simulink model "SingleLeg_R2013a"  (R2013a)
settings: Solver=FixedStepDiscrete  StartTime=0.0  StopTime=inf  FixedStep=0.001  RelTol=1e-3
libraries: xpcethercatlib x30, dspswit3 x1
settings Model: BufferReuse=off  Creator=bgbuss  LastModifiedBy=bgbuss
settings OptimizationCC: BlockReduction=off  OptimizeBlockIOStorage=off  BufferReuse=off  ExpressionFolding=off  LocalBlockOutputs=off
settings DebuggingCC: UnderspecifiedInitializationDetection=Simplified
settings HardwareCC: ProdIntDivRoundTo=Zero  ProdEndianess=LittleEndian  ProdHWDeviceType=Generic->32-bit x86 compatible
settings RTWCC: SystemTargetFile=xpctarget.tlc  TemplateMakefile=xpc_default_tmf  Description=xPC Target  ProcessScript=xpctarget_make_rtw_hook  RTWCompilerOptimization=On
settings CodeAppCC: MATLABSourceComments=on
settings xpcTargetCC: TargetFcnLib=ansi_tfl_table_tmw.mat  CodeReplacementLibrary=XPC_BLAS  ParMdlRefBuildCompliant=on  ConcurrentExecutionCompliant=on  CombineSignalStateStructs=off  MATLABClassNameForMDSCustomization=xpcAperiodicCustomization  GRTInterface=on  GenerateAllocFcn=off  RL32LogBufSizeModifier=100000000  xPCTaskExecutionProfile=off  xPCRL32EventNumber=5000  xPCisModelTimeout=off  xPCModelTimeoutSecs=20  xPCLoadParamSetFile=off  xPCConcurrentTasks=off  xPCEnableSFAnimation=off

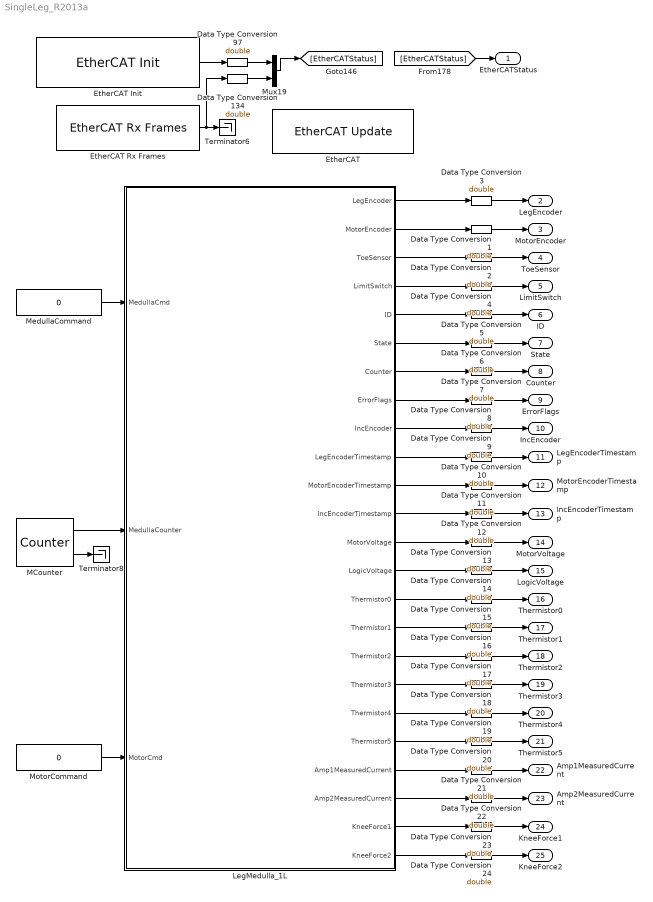
== system SingleLeg_R2013a ==
  Data Type Conversion{1..24,97,134} (26 alike) : DataTypeConversion  OutDataTypeStr=double
  EtherCAT : xpcethercatlib/EtherCAT Update   Priority=4  device_id=0  task_id_list=[1]  task_rates=[1]  task_priorities=[1500]
  "EtherCAT Init " : xpcethercatlib/EtherCAT Init   Priority=0  config_file='SingleLeg-eni.xml'  device_id=0  pci_bus=10  pci_slot=0  enaDC=on  errRptLevel=0  sample_time=-1
  EtherCAT Rx Frames : xpcethercatlib/EtherCAT Rx Frames   Priority=1  device_id=0  sample_time=0
  LegMedulla_1L : Subsystem
  MCounter : dspswit3/Counter  Direction=Up  CountEvent=Free running  CounterSize=User defined  MaxCount=65535  InitialCount=0  Output=Count and Hit  HitValue=32  ResetInput=off  SamplesPerFrame=1  Ts=.001  CntDtype=double  HitDtype=Logical
  MedullaCommand : Constant  Value=0
  MotorCommand : Constant  Value=0
  Mux19 : Mux  Inputs=2
  Terminator6 : Terminator
  Terminator8 : Terminator
  EtherCATStatus : Outport
  LegEncoder : Outport  Port=2
  MotorEncoder : Outport  Port=3
  ToeSensor : Outport  Port=4
  LimitSwitch : Outport  Port=5
  ID : Outport  Port=6
  State : Outport  Port=7
  Counter : Outport  Port=8
  ErrorFlags : Outport  Port=9
  IncEncoder : Outport  Port=10
  LegEncoderTimestamp : Outport  Port=11
  MotorEncoderTimestamp : Outport  Port=12
  IncEncoderTimestamp : Outport  Port=13
  MotorVoltage : Outport  Port=14
  LogicVoltage : Outport  Port=15
  Thermistor0 : Outport  Port=16
  Thermistor1 : Outport  Port=17
  Thermistor2 : Outport  Port=18
  Thermistor3 : Outport  Port=19
  Thermistor4 : Outport  Port=20
  Thermistor5 : Outport  Port=21
  Amp1MeasuredCurrent : Outport  Port=22
  Amp2MeasuredCurrent : Outport  Port=23
  KneeForce1 : Outport  Port=24
  KneeForce2 : Outport  Port=25
  wires:
  Data Type Conversion3/1 -> LegEncoder/1
  [EtherCATStatus] -> EtherCATStatus/1
  Mux19/1 -> [EtherCATStatus]
  "EtherCAT Init "/1 -> Data Type Conversion97/1
  LegMedulla_1L/2(MotorEncoder) -> Data Type Conversion1/1
  LegMedulla_1L/3(ToeSensor) -> Data Type Conversion2/1
  LegMedulla_1L/4(LimitSwitch) -> Data Type Conversion4/1
  LegMedulla_1L/5(ID) -> Data Type Conversion5/1
  LegMedulla_1L/6(State) -> Data Type Conversion6/1
  LegMedulla_1L/7(Counter) -> Data Type Conversion7/1
  LegMedulla_1L/8(ErrorFlags) -> Data Type Conversion8/1
  LegMedulla_1L/9(IncEncoder) -> Data Type Conversion9/1
  LegMedulla_1L/10(LegEncoderTimestamp) -> Data Type Conversion10/1
  LegMedulla_1L/11(MotorEncoderTimestamp) -> Data Type Conversion11/1
  LegMedulla_1L/12(IncEncoderTimestamp) -> Data Type Conversion12/1
  LegMedulla_1L/13(MotorVoltage) -> Data Type Conversion13/1
  LegMedulla_1L/14(LogicVoltage) -> Data Type Conversion14/1
  LegMedulla_1L/15(Thermistor0) -> Data Type Conversion15/1
  LegMedulla_1L/16(Thermistor1) -> Data Type Conversion16/1
  LegMedulla_1L/17(Thermistor2) -> Data Type Conversion17/1
  LegMedulla_1L/18(Thermistor3) -> Data Type Conversion18/1
  LegMedulla_1L/19(Thermistor4) -> Data Type Conversion19/1
  LegMedulla_1L/20(Thermistor5) -> Data Type Conversion20/1
  LegMedulla_1L/21(Amp1MeasuredCurrent) -> Data Type Conversion21/1
  LegMedulla_1L/22(Amp2MeasuredCurrent) -> Data Type Conversion22/1
  LegMedulla_1L/23(KneeForce1) -> Data Type Conversion23/1
  LegMedulla_1L/24(KneeForce2) -> Data Type Conversion24/1
  EtherCAT Rx Frames/1 -> Data Type Conversion134/1, Terminator6/1
  MCounter/2 -> Terminator8/1
  LegMedulla_1L/1(LegEncoder) -> Data Type Conversion3/1
  Data Type Conversion5/1 -> ID/1
  Data Type Conversion6/1 -> State/1
  Data Type Conversion7/1 -> Counter/1
  Data Type Conversion8/1 -> ErrorFlags/1
  Data Type Conversion9/1 -> IncEncoder/1
  Data Type Conversion10/1 -> LegEncoderTimestamp/1
  Data Type Conversion11/1 -> MotorEncoderTimestamp/1
  Data Type Conversion12/1 -> IncEncoderTimestamp/1
  Data Type Conversion13/1 -> MotorVoltage/1
  Data Type Conversion14/1 -> LogicVoltage/1
  Data Type Conversion15/1 -> Thermistor0/1
  Data Type Conversion16/1 -> Thermistor1/1
  Data Type Conversion17/1 -> Thermistor2/1
  Data Type Conversion18/1 -> Thermistor3/1
  Data Type Conversion19/1 -> Thermistor4/1
  Data Type Conversion20/1 -> Thermistor5/1
  Data Type Conversion21/1 -> Amp1MeasuredCurrent/1
  Data Type Conversion22/1 -> Amp2MeasuredCurrent/1
  Data Type Conversion23/1 -> KneeForce1/1
  Data Type Conversion24/1 -> KneeForce2/1
  MCounter/1 -> LegMedulla_1L/2(MedullaCounter)
  MedullaCommand/1 -> LegMedulla_1L/1(MedullaCmd)
  MotorCommand/1 -> LegMedulla_1L/3(MotorCmd)
  Data Type Conversion2/1 -> ToeSensor/1
  Data Type Conversion4/1 -> LimitSwitch/1
  Data Type Conversion1/1 -> MotorEncoder/1
  Data Type Conversion97/1 -> Mux19/1
  Data Type Conversion134/1 -> Mux19/2

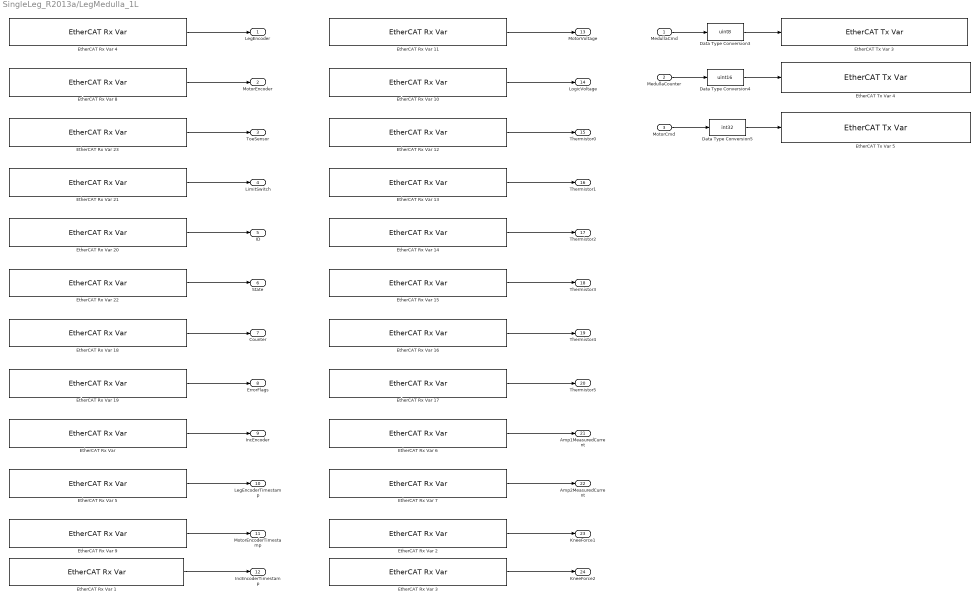
== system SingleLeg_R2013a/LegMedulla_1L ==
  MedullaCmd : Inport
  MedullaCounter : Inport  Port=2
  MotorCmd : Inport  Port=3
  Data Type Conversion3 : DataTypeConversion  OutDataTypeStr=uint8
  Data Type Conversion4 : DataTypeConversion  OutDataTypeStr=uint16
  Data Type Conversion5 : DataTypeConversion  OutDataTypeStr=int32
  "EtherCAT Rx Var " : xpcethercatlib/EtherCAT Rx Var   Priority=2  sig_name=Box 1 (ATRIAS 2.1 Leg (Medulla 1.5)).Incremental Encoder.Incremental Encoder  sig_offset=744  sig_type=uint16  type_size=16  sig_dim=1  device_id=0  sample_time=0.001000
  EtherCAT Rx Var 1 : xpcethercatlib/EtherCAT Rx Var   Priority=2  sig_name=Box 1 (ATRIAS 2.1 Leg (Medulla 1.5)).Incremental Encoder.Incremental Encoder Timestamp  sig_offset=760  sig_type=uint16  type_size=16  sig_dim=1  device_id=0  sample_time=0.001000
  EtherCAT Rx Var 10 : xpcethercatlib/EtherCAT Rx Var   Priority=2  sig_name=Box 1 (ATRIAS 2.1 Leg (Medulla 1.5)).Power.Logic Voltage  sig_offset=792  sig_type=uint16  type_size=16  sig_dim=1  device_id=0  sample_time=0.001000
  EtherCAT Rx Var 11 : xpcethercatlib/EtherCAT Rx Var   Priority=2  sig_name=Box 1 (ATRIAS 2.1 Leg (Medulla 1.5)).Power.Motor Voltage  sig_offset=776  sig_type=uint16  type_size=16  sig_dim=1  device_id=0  sample_time=0.001000
  EtherCAT Rx Var 12 : xpcethercatlib/EtherCAT Rx Var   Priority=2  sig_name=Box 1 (ATRIAS 2.1 Leg (Medulla 1.5)).Thermistors.Thermistor 0  sig_offset=808  sig_type=uint16  type_size=16  sig_dim=1  device_id=0  sample_time=0.001000
  EtherCAT Rx Var 13 : xpcethercatlib/EtherCAT Rx Var   Priority=2  sig_name=Box 1 (ATRIAS 2.1 Leg (Medulla 1.5)).Thermistors.Thermistor 1  sig_offset=824  sig_type=uint16  type_size=16  sig_dim=1  device_id=0  sample_time=0.001000
  EtherCAT Rx Var 14 : xpcethercatlib/EtherCAT Rx Var   Priority=2  sig_name=Box 1 (ATRIAS 2.1 Leg (Medulla 1.5)).Thermistors.Thermistor 2  sig_offset=840  sig_type=uint16  type_size=16  sig_dim=1  device_id=0  sample_time=0.001000
  EtherCAT Rx Var 15 : xpcethercatlib/EtherCAT Rx Var   Priority=2  sig_name=Box 1 (ATRIAS 2.1 Leg (Medulla 1.5)).Thermistors.Thermistor 3  sig_offset=856  sig_type=uint16  type_size=16  sig_dim=1  device_id=0  sample_time=0.001000
  EtherCAT Rx Var 16 : xpcethercatlib/EtherCAT Rx Var   Priority=2  sig_name=Box 1 (ATRIAS 2.1 Leg (Medulla 1.5)).Thermistors.Thermistor 4  sig_offset=872  sig_type=uint16  type_size=16  sig_dim=1  device_id=0  sample_time=0.001000
  EtherCAT Rx Var 17 : xpcethercatlib/EtherCAT Rx Var   Priority=2  sig_name=Box 1 (ATRIAS 2.1 Leg (Medulla 1.5)).Thermistors.Thermistor 5  sig_offset=888  sig_type=uint16  type_size=16  sig_dim=1  device_id=0  sample_time=0.001000
  EtherCAT Rx Var 18 : xpcethercatlib/EtherCAT Rx Var   Priority=2  sig_name=Box 1 (ATRIAS 2.1 Leg (Medulla 1.5)).uController Status.Counter  sig_offset=608  sig_type=uint8  type_size=8  sig_dim=1  device_id=0  sample_time=0.001000
  EtherCAT Rx Var 19 : xpcethercatlib/EtherCAT Rx Var   Priority=2  sig_name=Box 1 (ATRIAS 2.1 Leg (Medulla 1.5)).uController Status.Error Flags  sig_offset=616  sig_type=uint8  type_size=8  sig_dim=1  device_id=0  sample_time=0.001000
  EtherCAT Rx Var 2 : xpcethercatlib/EtherCAT Rx Var   Priority=2  sig_name=Box 1 (ATRIAS 2.1 Leg (Medulla 1.5)).Knee Force.Knee Force 1  sig_offset=936  sig_type=uint16  type_size=16  sig_dim=1  device_id=0  sample_time=0.001000
  EtherCAT Rx Var 20 : xpcethercatlib/EtherCAT Rx Var   Priority=2  sig_name=Box 1 (ATRIAS 2.1 Leg (Medulla 1.5)).uController Status.ID  sig_offset=592  sig_type=uint8  type_size=8  sig_dim=1  device_id=0  sample_time=0.001000
  EtherCAT Rx Var 21 : xpcethercatlib/EtherCAT Rx Var   Priority=2  sig_name=Box 1 (ATRIAS 2.1 Leg (Medulla 1.5)).uController Status.Limit Switch  sig_offset=624  sig_type=uint8  type_size=8  sig_dim=1  device_id=0  sample_time=0.001000
  EtherCAT Rx Var 22 : xpcethercatlib/EtherCAT Rx Var   Priority=2  sig_name=Box 1 (ATRIAS 2.1 Leg (Medulla 1.5)).uController Status.State  sig_offset=600  sig_type=uint8  type_size=8  sig_dim=1  device_id=0  sample_time=0.001000
  EtherCAT Rx Var 23 : xpcethercatlib/EtherCAT Rx Var   Priority=2  sig_name=Box 1 (ATRIAS 2.1 Leg (Medulla 1.5)).uController Status.Toe Sensor  sig_offset=632  sig_type=uint16  type_size=16  sig_dim=1  device_id=0  sample_time=0.001000
  EtherCAT Rx Var 3 : xpcethercatlib/EtherCAT Rx Var   Priority=2  sig_name=Box 1 (ATRIAS 2.1 Leg (Medulla 1.5)).Knee Force.Knee Force 2  sig_offset=952  sig_type=uint16  type_size=16  sig_dim=1  device_id=0  sample_time=0.001000
  EtherCAT Rx Var 4 : xpcethercatlib/EtherCAT Rx Var   Priority=2  sig_name=Box 1 (ATRIAS 2.1 Leg (Medulla 1.5)).Leg Encoder.Leg Encoder  sig_offset=696  sig_type=uint32  type_size=32  sig_dim=1  device_id=0  sample_time=0.001000
  EtherCAT Rx Var 5 : xpcethercatlib/EtherCAT Rx Var   Priority=2  sig_name=Box 1 (ATRIAS 2.1 Leg (Medulla 1.5)).Leg Encoder.Leg Encoder Timestamp  sig_offset=728  sig_type=uint16  type_size=16  sig_dim=1  device_id=0  sample_time=0.001000
  EtherCAT Rx Var 6 : xpcethercatlib/EtherCAT Rx Var   Priority=2  sig_name=Box 1 (ATRIAS 2.1 Leg (Medulla 1.5)).Measured Current.Amp 1 Measured Current  sig_offset=904  sig_type=int16  type_size=16  sig_dim=1  device_id=0  sample_time=0.001000
  EtherCAT Rx Var 7 : xpcethercatlib/EtherCAT Rx Var   Priority=2  sig_name=Box 1 (ATRIAS 2.1 Leg (Medulla 1.5)).Measured Current.Amp 2 Measured Current  sig_offset=920  sig_type=int16  type_size=16  sig_dim=1  device_id=0  sample_time=0.001000
  EtherCAT Rx Var 8 : xpcethercatlib/EtherCAT Rx Var   Priority=2  sig_name=Box 1 (ATRIAS 2.1 Leg (Medulla 1.5)).Motor Encoder.Motor Encoder  sig_offset=648  sig_type=uint32  type_size=32  sig_dim=1  device_id=0  sample_time=0.001000
  EtherCAT Rx Var 9 : xpcethercatlib/EtherCAT Rx Var   Priority=2  sig_name=Box 1 (ATRIAS 2.1 Leg (Medulla 1.5)).Motor Encoder.Motor Encoder Timestamp  sig_offset=680  sig_type=uint16  type_size=16  sig_dim=1  device_id=0  sample_time=0.001000
  EtherCAT Tx Var 3 : xpcethercatlib/EtherCAT Tx Var   Priority=3  sig_name=Box 1 (ATRIAS 2.1 Leg (Medulla 1.5)).uControllerInput.Command  sig_offset=592  sig_type=uint8  type_size=8  sig_dim=1  device_id=0  sample_time=0.001000
  EtherCAT Tx Var 4 : xpcethercatlib/EtherCAT Tx Var   Priority=3  sig_name=Box 1 (ATRIAS 2.1 Leg (Medulla 1.5)).uControllerInput.Counter  sig_offset=600  sig_type=uint16  type_size=16  sig_dim=1  device_id=0  sample_time=0.001000
  EtherCAT Tx Var 5 : xpcethercatlib/EtherCAT Tx Var   Priority=3  sig_name=Box 1 (ATRIAS 2.1 Leg (Medulla 1.5)).uControllerInput.Motor Current  sig_offset=616  sig_type=int32  type_size=32  sig_dim=1  device_id=0  sample_time=0.001000
  LegEncoder : Outport
  MotorEncoder : Outport  Port=2
  ToeSensor : Outport  Port=3
  LimitSwitch : Outport  Port=4
  ID : Outport  Port=5
  State : Outport  Port=6
  Counter : Outport  Port=7
  ErrorFlags : Outport  Port=8
  IncEncoder : Outport  Port=9
  LegEncoderTimestamp : Outport  Port=10
  MotorEncoderTimestamp : Outport  Port=11
  IncEncoderTimestamp : Outport  Port=12
  MotorVoltage : Outport  Port=13
  LogicVoltage : Outport  Port=14
  Thermistor0 : Outport  Port=15
  Thermistor1 : Outport  Port=16
  Thermistor2 : Outport  Port=17
  Thermistor3 : Outport  Port=18
  Thermistor4 : Outport  Port=19
  Thermistor5 : Outport  Port=20
  Amp1MeasuredCurrent : Outport  Port=21
  Amp2MeasuredCurrent : Outport  Port=22
  KneeForce1 : Outport  Port=23
  KneeForce2 : Outport  Port=24
  wires:
  Data Type Conversion3/1 -> EtherCAT Tx Var 3/1
  Data Type Conversion4/1 -> EtherCAT Tx Var 4/1
  Data Type Conversion5/1 -> EtherCAT Tx Var 5/1
  "EtherCAT Rx Var "/1 -> IncEncoder/1
  EtherCAT Rx Var 1/1 -> IncEncoderTimestamp/1
  EtherCAT Rx Var 2/1 -> KneeForce1/1
  EtherCAT Rx Var 3/1 -> KneeForce2/1
  EtherCAT Rx Var 4/1 -> LegEncoder/1
  EtherCAT Rx Var 5/1 -> LegEncoderTimestamp/1
  EtherCAT Rx Var 6/1 -> Amp1MeasuredCurrent/1
  EtherCAT Rx Var 7/1 -> Amp2MeasuredCurrent/1
  EtherCAT Rx Var 8/1 -> MotorEncoder/1
  EtherCAT Rx Var 9/1 -> MotorEncoderTimestamp/1
  EtherCAT Rx Var 10/1 -> LogicVoltage/1
  EtherCAT Rx Var 11/1 -> MotorVoltage/1
  EtherCAT Rx Var 12/1 -> Thermistor0/1
  EtherCAT Rx Var 13/1 -> Thermistor1/1
  EtherCAT Rx Var 14/1 -> Thermistor2/1
  EtherCAT Rx Var 15/1 -> Thermistor3/1
  EtherCAT Rx Var 16/1 -> Thermistor4/1
  EtherCAT Rx Var 17/1 -> Thermistor5/1
  EtherCAT Rx Var 18/1 -> Counter/1
  EtherCAT Rx Var 19/1 -> ErrorFlags/1
  EtherCAT Rx Var 20/1 -> ID/1
  EtherCAT Rx Var 21/1 -> LimitSwitch/1
  EtherCAT Rx Var 22/1 -> State/1
  EtherCAT Rx Var 23/1 -> ToeSensor/1
  MedullaCmd/1 -> Data Type Conversion3/1
  MedullaCounter/1 -> Data Type Conversion4/1
  MotorCmd/1 -> Data Type Conversion5/1
